simulink library "SoftRobotics"  (R2024a)
settings: Solver=VariableStepAuto  StartTime=0.0  StopTime=10.0  RelTol=1e-3
undefined symbols (not defined in the file or in its folder): bt, sr
settings Model: Creator=pietro  LastModifiedBy=pietro
settings OptimizationCC: ReuseModelBlockBuffer=off
settings RTWCC: GPUComputeCapability=3.5

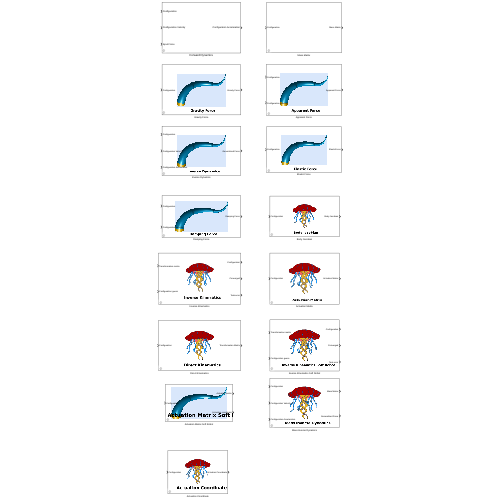
[thumbnail: Simulink's stored preview of the top-level diagram]
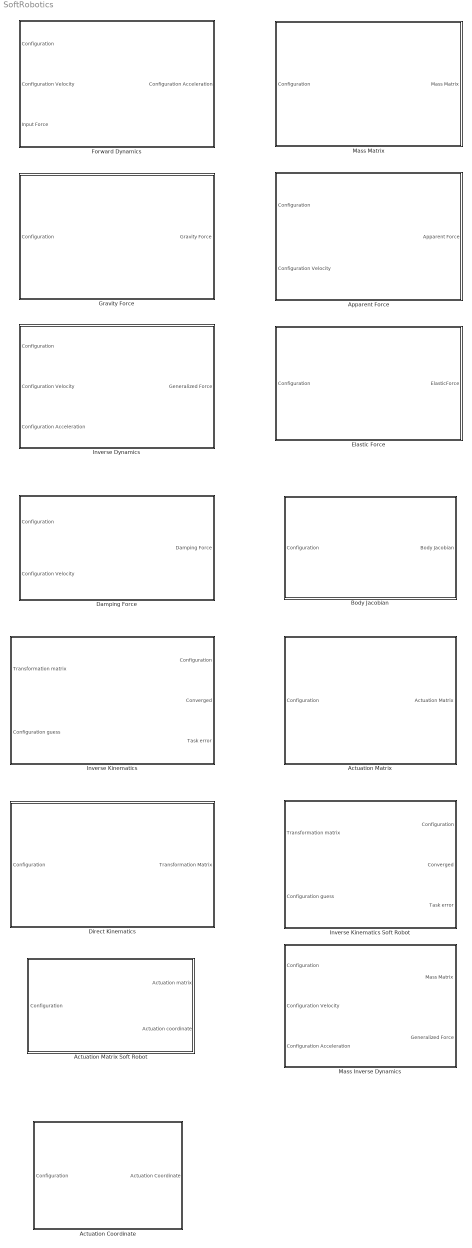
== system SoftRobotics ==
  Actuation Coordinate : Subsystem  mask{robotModel=bt, SimulateUsing=Code generation}
      mask prompts: SimulateUsing "SystemBlock:MATLABSystem:SimulateUsing"
      mask init:
      | %Get the robot representation as a struct (required for code generation)
      | Tree        = evalin('base', get_param(gcb, 'robotModel'));
      | robotStruct = TreeStructConverter.ObjectToStruct(Tree);
      | %Set the struct as a parameter of the underlying block
      | set_param([gcb '/' 'ActuationCoordinateSystem'], 'RobotStruct', 'robotStruct');
      mask TypeOptions SimulateUsing: ActuationCoordinateSystem/SimulateUsing
      mask DialogControl SimulateUsing Prompt: Simulate using:
      mask DialogControl SimulateUsing Tooltip: SystemBlock:MATLABSystem:SimulateUsingDescription
  Actuation Matrix : Subsystem  mask{robotModel=bt, SimulateUsing=Code generation}
      mask prompts: SimulateUsing "SystemBlock:MATLABSystem:SimulateUsing"
      mask init:
      | %Get the robot representation as a struct (required for code generation)
      | Tree        = evalin('base', get_param(gcb, 'robotModel'));
      | robotStruct = TreeStructConverter.ObjectToStruct(Tree);
      | %Set the struct as a parameter of the underlying block
      | set_param([gcb '/' 'ActuationMatrixSystem'], 'RobotStruct', 'robotStruct');
      mask TypeOptions SimulateUsing: ActuationMatrixSystem/SimulateUsing
      mask DialogControl SimulateUsing Prompt: Simulate using:
      mask DialogControl SimulateUsing Tooltip: SystemBlock:MATLABSystem:SimulateUsingDescription
  Actuation Matrix Soft Robot : Subsystem  mask{robotModel=sr, SimulateUsing=Code generation}
      mask prompts: SimulateUsing "SystemBlock:MATLABSystem:SimulateUsing"
      mask init:
      | %Get the robot representation as a struct (required for code generation)
      | Tree        = evalin('base', get_param(gcb, 'robotModel'));
      | robotStruct = SoftRobotStructConverter.ObjectToStruct(Tree);
      | %Set the struct as a parameter of the underlying block
      | set_param([gcb '/' 'ActuationMatrixSystemSoftRobot'], 'SoftRobotStruct', 'robotStruct');
      mask TypeOptions SimulateUsing: ActuationMatrixSystemSoftRobot/SimulateUsing
      mask DialogControl SimulateUsing Prompt: Simulate using:
      mask DialogControl SimulateUsing Tooltip: SystemBlock:MATLABSystem:SimulateUsingDescription
  Apparent Force : Subsystem  mask{robotModel=bt, SimulateUsing=Code generation}
      mask prompts: robotModel "Robot Model"; SimulateUsing "SystemBlock:MATLABSystem:SimulateUsing"
      mask init:
      | %Get the robot representation as a struct (required for code generation)
      | Tree = evalin('base', get_param(gcb, 'RobotModel'));
      | robotStruct = TreeStructConverter.ObjectToStruct(Tree);
      | %Set the struct as a parameter of the underlying block
      | set_param([gcb '/' 'ApparentForceSystem'], 'RobotStruct', 'robotStruct');
      mask TypeOptions SimulateUsing: ApparentForceSystem/SimulateUsing
      mask DialogControl SimulateUsing Prompt: Simulate using:
      mask DialogControl SimulateUsing Tooltip: SystemBlock:MATLABSystem:SimulateUsingDescription
  Body Jacobian : Subsystem  mask{robotModel=bt, SimulateUsing=Code generation, BodyIndexes=0}
      mask prompts: robotModel "Robot Model"; SimulateUsing "SystemBlock:MATLABSystem:SimulateUsing"; BodyIndexes "Indexes of the bodies for which the Jacobian is to be evaluated:"
      mask init:
      | %Get the robot representation as a struct (required for code generation)
      | Tree        = evalin('base', get_param(gcb, 'robotModel'));
      | robotStruct = TreeStructConverter.ObjectToStruct(Tree);
      | 
      | % Get the length of the body index vector
      | bodyIdx    = evalin('base', get_param(gcb, 'BodyIndexes'));
      | bodyLength = length(bodyIdx);
      | 
      | %Set the struct as a parameter of the underlying block
      | set_param([gcb '/' 'BodyJacobianSystem'], 'RobotStruct', 'robotStruct', 'BodyIndexesLength', 'bodyLength');
      mask TypeOptions SimulateUsing: BodyJacobianSystem/SimulateUsing
      mask TypeOptions BodyIndexes: BodyJacobianSystem/BodyIndexes
      mask DialogControl SimulateUsing Prompt: Simulate using:
      mask DialogControl SimulateUsing Tooltip: SystemBlock:MATLABSystem:SimulateUsingDescription
  Damping Force : Subsystem  mask{robotModel=bt, SimulateUsing=Code generation}
      mask prompts: robotModel "Robot Model"; SimulateUsing "SystemBlock:MATLABSystem:SimulateUsing"
      mask init:
      | %Get the robot representation as a struct (required for code generation)
      | Tree = evalin('base', get_param(gcb, 'RobotModel'));
      | robotStruct = TreeStructConverter.ObjectToStruct(Tree);
      | %Set the struct as a parameter of the underlying block
      | set_param([gcb '/' 'DampingForceSystem'], 'RobotStruct', 'robotStruct');
      mask TypeOptions SimulateUsing: DampingForceSystem/SimulateUsing
      mask DialogControl SimulateUsing Prompt: Simulate using:
      mask DialogControl SimulateUsing Tooltip: SystemBlock:MATLABSystem:SimulateUsingDescription
  Direct Kinematics : Subsystem  mask{robotModel=bt, SimulateUsing=Code generation, BodyIndexes=0}
      mask prompts: SimulateUsing "SystemBlock:MATLABSystem:SimulateUsing"; BodyIndexes "Indexed of the bodies for which the direct kinematics has to be:"
      mask init:
      | %Get the robot representation as a struct (required for code generation)
      | Tree        = evalin('base', get_param(gcb, 'robotModel'));
      | robotStruct = TreeStructConverter.ObjectToStruct(Tree);
      | 
      | % Get the length of the body index vector
      | bodyIdx    = evalin('base', get_param(gcb, 'BodyIndexes'));
      | bodyLength = length(bodyIdx);
      | 
      | %Set the struct as a parameter of the underlying block
      | set_param([gcb '/' 'DirectKinematicsSystem'], 'RobotStruct', 'robotStruct', 'BodyIndexesLength', 'bodyLength');
      mask TypeOptions SimulateUsing: DirectKinematicsSystem/SimulateUsing
      mask TypeOptions BodyIndexes: DirectKinematicsSystem/BodyIndexes
      mask DialogControl SimulateUsing Prompt: Simulate using:
      mask DialogControl SimulateUsing Tooltip: SystemBlock:MATLABSystem:SimulateUsingDescription
  Elastic Force : Subsystem  mask{robotModel=bt, SimulateUsing=Code generation}
      mask prompts: robotModel "Robot Model"; SimulateUsing "SystemBlock:MATLABSystem:SimulateUsing"
      mask init:
      | %Get the robot representation as a struct (required for code generation)
      | Tree = evalin('base', get_param(gcb, 'RobotModel'));
      | robotStruct = TreeStructConverter.ObjectToStruct(Tree);
      | %Set the struct as a parameter of the underlying block
      | set_param([gcb '/' 'ElasticForceSystem'], 'RobotStruct', 'robotStruct');
      mask TypeOptions SimulateUsing: ElasticForceSystem/SimulateUsing
      mask DialogControl SimulateUsing Prompt: Simulate using:
      mask DialogControl SimulateUsing Tooltip: SystemBlock:MATLABSystem:SimulateUsingDescription
  Forward Dynamics : Subsystem  mask{RobotModel=bt, SimulateUsing=Code generation}
      mask prompts: RobotModel "Robot model"; SimulateUsing "Simulate using:"
      mask init:
      | %TODO: Add various checks that the paramter is correct.
      | 
      | %Get the robot representation as a struct (required for code generation)
      | Tree = evalin('base', get_param(gcb, 'RobotModel'));
      | robotStruct = TreeStructConverter.ObjectToStruct(Tree);
      | %Set the struct as a parameter of the underlying block
      | set_param([gcb '/' 'ForwardDynamicsSystem'], 'RobotStruct', 'robotStruct');
      mask TypeOptions SimulateUsing: ForwardDynamicsSystem/SimulateUsing
      mask DialogControl DescTextVar Prompt: Implementazione delle forward dynamics
      mask DialogControl SimulateUsing Tooltip: SystemBlock:MATLABSystem:SimulateUsingDescription
  Gravity Force : Subsystem  mask{robotModel=bt, SimulateUsing=Code generation}
      mask prompts: robotModel "Robot Model"; SimulateUsing "SystemBlock:MATLABSystem:SimulateUsing"
      mask init:
      | %Get the robot representation as a struct (required for code generation)
      | Tree = evalin('base', get_param(gcb, 'RobotModel'));
      | robotStruct = TreeStructConverter.ObjectToStruct(Tree);
      | %Set the struct as a parameter of the underlying block
      | set_param([gcb '/' 'GravityForceSystem'], 'RobotStruct', 'robotStruct');
      mask TypeOptions SimulateUsing: GravityForceSystem/SimulateUsing
      mask DialogControl SimulateUsing Prompt: Simulate using:
      mask DialogControl SimulateUsing Tooltip: SystemBlock:MATLABSystem:SimulateUsingDescription
  Inverse Dynamics : Subsystem  mask{robotModel=bt, SimulateUsing=Code generation, EvaluateExternalForces=on}
      mask prompts: robotModel "Robot Model"; SimulateUsing "SystemBlock:MATLABSystem:SimulateUsing"; EvaluateExternalForces "Evaluate generalized external forces such as damping and elastic forces."
      mask init:
      | %Get the robot representation as a struct (required for code generation)
      | Tree = evalin('base', get_param(gcb, 'RobotModel'));
      | robotStruct = TreeStructConverter.ObjectToStruct(Tree);
      | %Set the struct as a parameter of the underlying block
      | set_param([gcb '/' 'InverseDynamicsSystem'], 'RobotStruct', 'robotStruct');
      mask TypeOptions SimulateUsing: InverseDynamicsSystem/SimulateUsing
      mask TypeOptions EvaluateExternalForces: InverseDynamicsSystem/EvaluateExternalForces
      mask DialogControl SimulateUsing Prompt: Simulate using:
      mask DialogControl SimulateUsing Tooltip: SystemBlock:MATLABSystem:SimulateUsingDescription
  Inverse Kinematics : Subsystem  mask{robotModel=bt, SimulateUsing=Code generation, BodyIndexes=1, MaximumNewtonIterations=4, TaskSpaceFlags=ones( 6, 1 )}
      mask prompts: robotModel "Robot Model"; SimulateUsing "SystemBlock:MATLABSystem:SimulateUsing"; BodyIndexes "Indexes of the bodies to consider in the inverse kinematics:"; MaximumNewtonIterations "Maximum number of Newton iterations:"; TaskSpaceFlags "Task space flags:"
      mask init:
      | %Get the robot representation as a struct (required for code generation)
      | Tree        = evalin('base', get_param(gcb, 'robotModel'));
      | robotStruct = TreeStructConverter.ObjectToStruct(Tree);
      | %Set the struct as a parameter of the underlying block
      | set_param([gcb '/' 'InverseKinematicsSystem'], 'RobotStruct', 'robotStruct');
      mask TypeOptions SimulateUsing: InverseKinematicsSystem/SimulateUsing
      mask TypeOptions BodyIndexes: InverseKinematicsSystem/BodyIndexes
      mask TypeOptions MaximumNewtonIterations: InverseKinematicsSystem/MaximumNewtonIterations
      mask TypeOptions TaskSpaceFlags: InverseKinematicsSystem/TaskSpaceFlags
      mask DialogControl SimulateUsing Prompt: Simulate using:
      mask DialogControl SimulateUsing Tooltip: SystemBlock:MATLABSystem:SimulateUsingDescription
  Inverse Kinematics Soft Robot : Subsystem  mask{robotModel=sr, SimulateUsing=Code generation, BodyPoints=0, MaximumNewtonIterations=4, TaskSpaceFlags=ones( 6, 1 ), AngularErrorThreshold=1e-3, LinearErrorThreshold=1e-2, UseGradientDescent=on, GradientDescentStepSize=1, ErrorWeight=1}
      mask prompts: robotModel "Soft Robot model"; SimulateUsing "SystemBlock:MATLABSystem:SimulateUsing"; BodyPoints "Points along the backbone to consider in the inverse kinematics:"; MaximumNewtonIterations "Maximum number of Newton iterations:"; TaskSpaceFlags "Task space flags:"; AngularErrorThreshold "Angular error threshold:"; LinearErrorThreshold "Linear error threshold:"; UseGradientDescent "Use Gradient Descent"; GradientDescentStepSize "Step size for the gradient descent:"; ErrorWeight "Weight for the error:"
      mask init:
      | %Get the robot representation as a struct (required for code generation)
      | Tree        = evalin('base', get_param(gcb, 'robotModel'));
      | robotStruct = SoftRobotStructConverter.ObjectToStruct(Tree);
      | %Set the struct as a parameter of the underlying block
      | set_param([gcb '/' 'InverseKinematicsSoftRobotSystem'], 'SoftRobotStruct', 'robotStruct');
      mask TypeOptions SimulateUsing: InverseKinematicsSoftRobotSystem/SimulateUsing
      mask TypeOptions BodyPoints: InverseKinematicsSoftRobotSystem/BodyPoints
      mask TypeOptions MaximumNewtonIterations: InverseKinematicsSoftRobotSystem/MaximumNewtonIterations
      mask TypeOptions TaskSpaceFlags: InverseKinematicsSoftRobotSystem/TaskSpaceFlags
      mask TypeOptions AngularErrorThreshold: InverseKinematicsSoftRobotSystem/AngularErrorThreshold
      mask TypeOptions LinearErrorThreshold: InverseKinematicsSoftRobotSystem/LinearErrorThreshold
      mask TypeOptions UseGradientDescent: InverseKinematicsSoftRobotSystem/UseGradientDescent
      mask Callback UseGradientDescent:
      | % Set the visibility of the terms
      |     p     = Simulink.Mask.get(gcb);
      |     paramUseGradientDescent = p.getParameter('UseGradientDescent');
      |     % Get the parameters that must not be visibile
      |     paramGradientDescentStepSize = p.getParameter('GradientDescentStepSize');
      |     %paramErrorWeight = p.getParameter('ErrorWeight');
      |     if strcmp(get_param(gcb, 'UseGradientDescent'), 'on')
      |         paramGradientDescentStepSize.Visible = 'on';
      |         %paramErrorWeight.Visible            = 'on';
      |     else
      |         paramGradientDescentStepSize.Visible = 'off';
      |         %paramErrorWeight.Visible            = 'off';
      |     end
      mask TypeOptions GradientDescentStepSize: InverseKinematicsSoftRobotSystem/GradientDescentStepSize
      mask TypeOptions ErrorWeight: InverseKinematicsSoftRobotSystem/ErrorWeight
      mask DialogControl SimulateUsing Prompt: Simulate using:
      mask DialogControl SimulateUsing Tooltip: SystemBlock:MATLABSystem:SimulateUsingDescription
  Mass Inverse Dynamics : Subsystem  mask{robotModel=bt, SimulateUsing=Code generation, EvaluateExternalForces=on}
      mask prompts: robotModel "Robot Model"; SimulateUsing "SystemBlock:MATLABSystem:SimulateUsing"; EvaluateExternalForces "Evaluate generalized external forces such as damping and elastic forces."
      mask init:
      | %Get the robot representation as a struct (required for code generation)
      | Tree = evalin('base', get_param(gcb, 'robotModel'));
      | robotStruct = TreeStructConverter.ObjectToStruct(Tree);
      | %Set the struct as a parameter of the underlying block
      | set_param([gcb '/' 'MassInverseDynamicsSystem'], 'RobotStruct', 'robotStruct');
      mask TypeOptions SimulateUsing: MassInverseDynamicsSystem/SimulateUsing
      mask TypeOptions EvaluateExternalForces: MassInverseDynamicsSystem/EvaluateExternalForces
      mask DialogControl SimulateUsing Prompt: Simulate using:
      mask DialogControl SimulateUsing Tooltip: SystemBlock:MATLABSystem:SimulateUsingDescription
  Mass Matrix : Subsystem  mask{RobotModel=bt, SimulateUsing=Code generation}
      mask prompts: RobotModel "Robot model"; SimulateUsing "SystemBlock:MATLABSystem:SimulateUsing"
      mask init:
      | %Get the robot representation as a struct (required for code generation)
      | Tree = evalin('base', get_param(gcb, 'RobotModel'));
      | robotStruct = TreeStructConverter.ObjectToStruct(Tree);
      | %Set the struct as a parameter of the underlying block
      | set_param([gcb '/' 'MassMatrixSystem'], 'RobotStruct', 'robotStruct');
      mask TypeOptions SimulateUsing: MassMatrixSystem/SimulateUsing
      mask DialogControl SimulateUsing Prompt: Simulate using:
      mask DialogControl SimulateUsing Tooltip: SystemBlock:MATLABSystem:SimulateUsingDescription

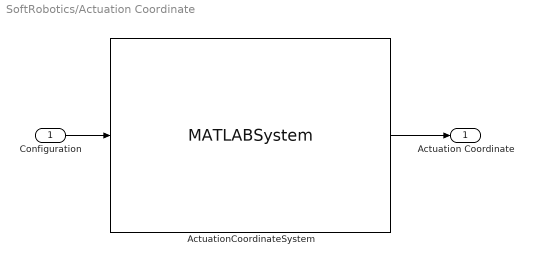
== system SoftRobotics/Actuation Coordinate ==
  Configuration : Inport
  ActuationCoordinateSystem : MATLABSystem  System=ActuationCoordinateSystem  RobotStruct=0  SimulateUsing=Code generation
      mask Type: ActuationCoordinateSystem
      mask Display:
      | disp('ActuationCoordinateSystem');
      | port_label('input',1,'q');
      | port_label('output',1,'y');
  Actuation Coordinate : Outport
  wires:
  Configuration/1 -> ActuationCoordinateSystem/1
  ActuationCoordinateSystem/1 -> Actuation Coordinate/1

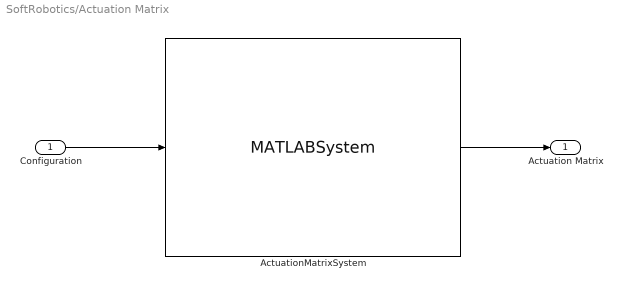
== system SoftRobotics/Actuation Matrix ==
  Configuration : Inport
  ActuationMatrixSystem : MATLABSystem  System=ActuationMatrixSystem  RobotStruct=0  SimulateUsing=Code generation
      mask Type: ActuationMatrixSystem
      mask Display:
      | disp('ActuationMatrixSystem');
      | port_label('input',1,'q');
      | port_label('output',1,'A');
  Actuation Matrix : Outport
  wires:
  ActuationMatrixSystem/1 -> Actuation Matrix/1
  Configuration/1 -> ActuationMatrixSystem/1

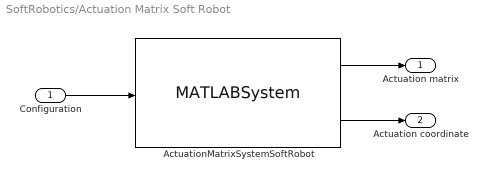
== system SoftRobotics/Actuation Matrix Soft Robot ==
  Configuration : Inport
  ActuationMatrixSystemSoftRobot : MATLABSystem  System=ActuationMatrixSystemSoftRobot  SoftRobotStruct=0  SimulateUsing=Code generation
      mask Type: ActuationMatrixSystemSoftRobot
      mask Display:
      | disp('ActuationMatrixSystemSoftRobot');
      | port_label('input',1,'q');
      | port_label('output',1,'A');
      | port_label('output',2,'y');
  Actuation matrix : Outport
  Actuation coordinate : Outport  Port=2
  wires:
  Configuration/1 -> ActuationMatrixSystemSoftRobot/1
  ActuationMatrixSystemSoftRobot/2 -> Actuation coordinate/1
  ActuationMatrixSystemSoftRobot/1 -> Actuation matrix/1

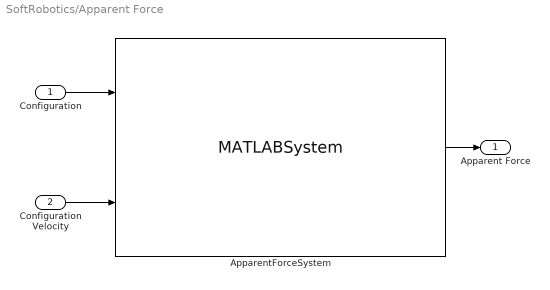
== system SoftRobotics/Apparent Force ==
  Configuration : Inport
  Configuration Velocity : Inport  Port=2
  ApparentForceSystem : MATLABSystem  System=ApparentForceSystem  RobotStruct=robotStruct  SimulateUsing=Code generation
      mask Type: ApparentForceSystem
      mask Display:
      | disp('ApparentForceSystem');
      | port_label('input',1,'q');
      | port_label('input',2,'dq');
      | port_label('output',1,'C');
  Apparent Force : Outport
  wires:
  Configuration Velocity/1 -> ApparentForceSystem/2
  ApparentForceSystem/1 -> Apparent Force/1
  Configuration/1 -> ApparentForceSystem/1

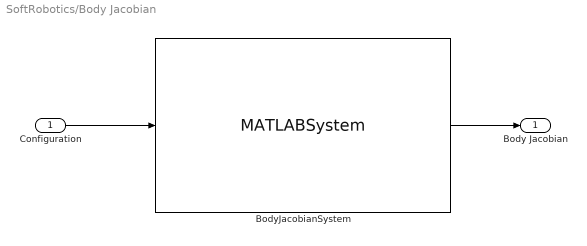
== system SoftRobotics/Body Jacobian ==
  Configuration : Inport
  BodyJacobianSystem : MATLABSystem  System=BodyJacobianSystem  RobotStruct=bt  BodyIndexes=BodyIndexes  BodyIndexesLength=[]  SimulateUsing=Code generation
      mask Type: BodyJacobianSystem
      mask Display:
      | disp('BodyJacobianSystem');
      | port_label('input',1,'q');
      | port_label('output',1,'J');
  Body Jacobian : Outport
  wires:
  Configuration/1 -> BodyJacobianSystem/1
  BodyJacobianSystem/1 -> Body Jacobian/1

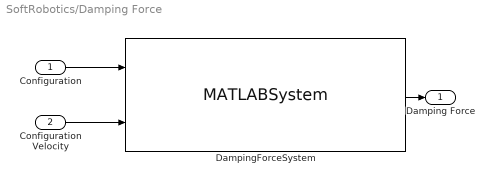
== system SoftRobotics/Damping Force ==
  Configuration : Inport
  Configuration Velocity : Inport  Port=2
  DampingForceSystem : MATLABSystem  System=DampingForceSystem  RobotStruct=robotStruct  SimulateUsing=Code generation
      mask Type: DampingForceSystem
      mask Display:
      | disp('DampingForceSystem');
      | port_label('input',1,'q');
      | port_label('input',2,'dq');
      | port_label('output',1,'D');
  Damping Force : Outport
  wires:
  Configuration/1 -> DampingForceSystem/1
  DampingForceSystem/1 -> Damping Force/1
  Configuration Velocity/1 -> DampingForceSystem/2

== system SoftRobotics/Direct Kinematics ==
  Configuration : Inport
  DirectKinematicsSystem : MATLABSystem  System=DirectKinematicsSystem  RobotStruct=0  BodyIndexes=BodyIndexes  BodyIndexesLength=0  SimulateUsing=Code generation
      mask Type: DirectKinematicsSystem
      mask Display:
      | disp('DirectKinematicsSystem');
      | port_label('input',1,'q');
      | port_label('output',1,'T');
  Transformation Matrix : Outport
  wires:
  DirectKinematicsSystem/1 -> Transformation Matrix/1
  Configuration/1 -> DirectKinematicsSystem/1

== system SoftRobotics/Elastic Force ==
  Configuration : Inport
  ElasticForceSystem : MATLABSystem  System=ElasticForceSystem  RobotStruct=robotStruct  SimulateUsing=Code generation
      mask Type: ElasticForceSystem
      mask Display:
      | disp('ElasticForceSystem');
      | port_label('input',1,'q');
      | port_label('output',1,'K');
  ElasticForce : Outport
  wires:
  Configuration/1 -> ElasticForceSystem/1
  ElasticForceSystem/1 -> ElasticForce/1

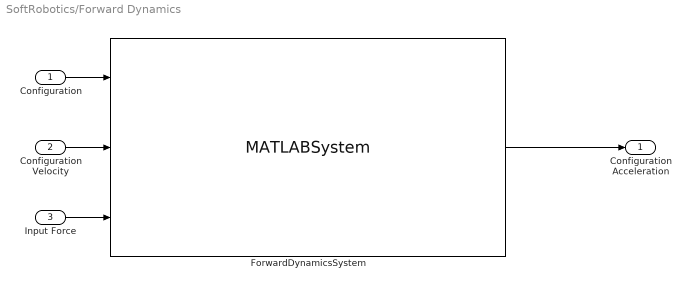
== system SoftRobotics/Forward Dynamics ==
  Configuration : Inport
  Configuration Velocity : Inport  Port=2
  Input Force : Inport  Port=3
  ForwardDynamicsSystem : MATLABSystem  System=ForwardDynamicsSystem  RobotStruct=robotStruct  SimulateUsing=Code generation
      mask Type: ForwardDynamicsSystem
      mask Display:
      | disp('ForwardDynamicsSystem');
      | port_label('input',1,'q');
      | port_label('input',2,'dq');
      | port_label('input',3,'u');
      | port_label('output',1,'ddq');
  Configuration Acceleration : Outport
  wires:
  Configuration/1 -> ForwardDynamicsSystem/1
  Configuration Velocity/1 -> ForwardDynamicsSystem/2
  Input Force/1 -> ForwardDynamicsSystem/3
  ForwardDynamicsSystem/1 -> Configuration Acceleration/1

== system SoftRobotics/Gravity Force ==
  Configuration : Inport
  GravityForceSystem : MATLABSystem  System=GravityForceSystem  RobotStruct=robotStruct  SimulateUsing=Code generation
      mask Type: GravityForceSystem
      mask Display:
      | disp('GravityForceSystem');
      | port_label('input',1,'q');
      | port_label('output',1,'G');
  Gravity Force : Outport
  wires:
  Configuration/1 -> GravityForceSystem/1
  GravityForceSystem/1 -> Gravity Force/1

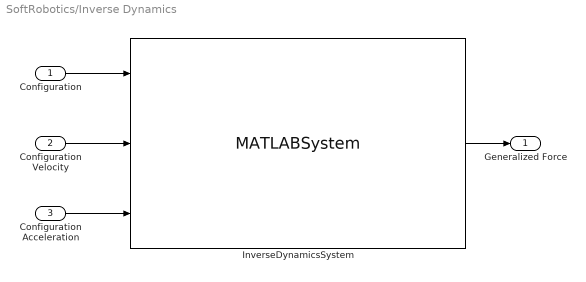
== system SoftRobotics/Inverse Dynamics ==
  Configuration : Inport
  Configuration Velocity : Inport  Port=2
  Configuration Acceleration : Inport  Port=3
  InverseDynamicsSystem : MATLABSystem  System=InverseDynamicsSystem  RobotStruct=robotStruct  EvaluateExternalForces=on  SimulateUsing=Code generation
      mask Type: InverseDynamicsSystem
      mask Display:
      | disp('InverseDynamicsSystem');
      | port_label('input',1,'q');
      | port_label('input',2,'dq');
      | port_label('input',3,'ddq');
      | port_label('output',1,'u');
  Generalized Force : Outport
  wires:
  Configuration Velocity/1 -> InverseDynamicsSystem/2
  InverseDynamicsSystem/1 -> Generalized Force/1
  Configuration/1 -> InverseDynamicsSystem/1
  Configuration Acceleration/1 -> InverseDynamicsSystem/3

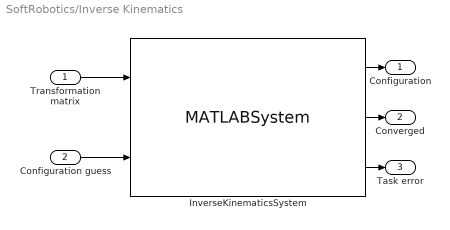
== system SoftRobotics/Inverse Kinematics ==
  Transformation matrix : Inport
  Configuration guess : Inport  Port=2
  InverseKinematicsSystem : MATLABSystem  System=InverseKinematicsSystem  RobotStruct=0  BodyIndexes=BodyIndexes  MaximumNewtonIterations=MaximumNewtonIterations  TaskSpaceFlags=TaskSpaceFlags  SimulateUsing=Code generation
      mask Type: InverseKinematicsSystem
      mask Display:
      | disp('InverseKinematicsSystem');
      | port_label('input',1,'T');
      | port_label('input',2,'q0');
      | port_label('output',1,'q');
      | port_label('output',2,'converged');
      | port_label('output',3,'e');
  Configuration : Outport
  Converged : Outport  Port=2
  Task error : Outport  Port=3
  wires:
  Configuration guess/1 -> InverseKinematicsSystem/2
  InverseKinematicsSystem/1 -> Configuration/1
  Transformation matrix/1 -> InverseKinematicsSystem/1
  InverseKinematicsSystem/2 -> Converged/1
  InverseKinematicsSystem/3 -> Task error/1

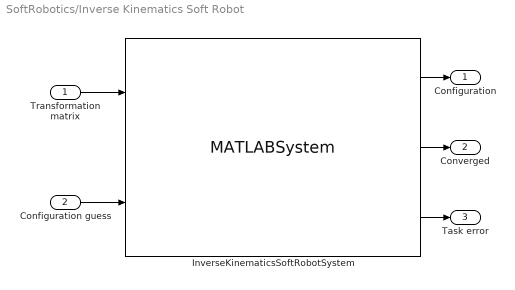
== system SoftRobotics/Inverse Kinematics Soft Robot ==
  Transformation matrix : Inport
  Configuration guess : Inport  Port=2
  InverseKinematicsSoftRobotSystem : MATLABSystem  System=InverseKinematicsSoftRobotSystem  SoftRobotStruct=0  BodyPoints=BodyPoints  MaximumNewtonIterations=MaximumNewtonIterations  TaskSpaceFlags=TaskSpaceFlags  AngularErrorThreshold=AngularErrorThreshold  LinearErrorThreshold=LinearErrorThreshold  UseGradientDescent=on  GradientDescentStepSize=GradientDescentStepSize  ErrorWeight=ErrorWeight  SimulateUsing=Code generation
      mask Type: InverseKinematicsSoftRobotSystem
      mask Display:
      | disp('InverseKinematicsSoftRobotSystem');
      | port_label('input',1,'T');
      | port_label('input',2,'q0');
      | port_label('output',1,'q');
      | port_label('output',2,'converged');
      | port_label('output',3,'e');
  Configuration : Outport
  Converged : Outport  Port=2
  Task error : Outport  Port=3
  wires:
  Configuration guess/1 -> InverseKinematicsSoftRobotSystem/2
  InverseKinematicsSoftRobotSystem/1 -> Configuration/1
  InverseKinematicsSoftRobotSystem/3 -> Task error/1
  Transformation matrix/1 -> InverseKinematicsSoftRobotSystem/1
  InverseKinematicsSoftRobotSystem/2 -> Converged/1

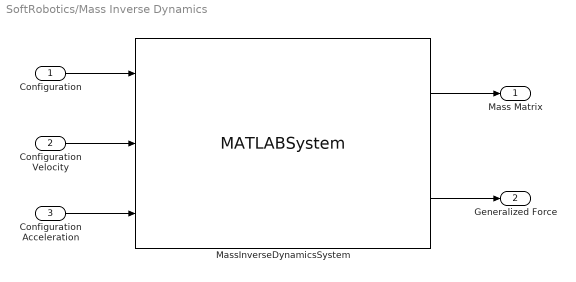
== system SoftRobotics/Mass Inverse Dynamics ==
  Configuration : Inport
  Configuration Velocity : Inport  Port=2
  Configuration Acceleration : Inport  Port=3
  MassInverseDynamicsSystem : MATLABSystem  System=MassInverseDynamicsSystem  RobotStruct=0  EvaluateExternalForces=on  SimulateUsing=Code generation
      mask Type: MassInverseDynamicsSystem
      mask Display:
      | disp('MassInverseDynamicsSystem');
      | port_label('input',1,'q');
      | port_label('input',2,'dq');
      | port_label('input',3,'ddq');
      | port_label('output',1,'M');
      | port_label('output',2,'tau');
  Mass Matrix : Outport
  Generalized Force : Outport  Port=2
  wires:
  Configuration Acceleration/1 -> MassInverseDynamicsSystem/3
  Configuration Velocity/1 -> MassInverseDynamicsSystem/2
  MassInverseDynamicsSystem/2 -> Generalized Force/1
  MassInverseDynamicsSystem/1 -> Mass Matrix/1
  Configuration/1 -> MassInverseDynamicsSystem/1

== system SoftRobotics/Mass Matrix ==
  Configuration : Inport
  MassMatrixSystem : MATLABSystem  System=MassMatrixSystem  RobotStruct=robotStruct  SimulateUsing=Code generation
      mask Type: MassMatrixSystem
      mask Display:
      | disp('MassMatrixSystem');
      | port_label('input',1,'q');
      | port_label('output',1,'M');
  Mass Matrix : Outport
  wires:
  Configuration/1 -> MassMatrixSystem/1
  MassMatrixSystem/1 -> Mass Matrix/1
